simulink library "Collector_EN12975_FlatPlate_CONF"  (R2013b)
settings: Solver=ode45  StartTime=0.0  StopTime=10.0  RelTol=1e-3
undefined symbols (not defined in the file): FPC
libraries: carnot x2
settings Model: Creator=lena.frank  LastModifiedBy=drhf

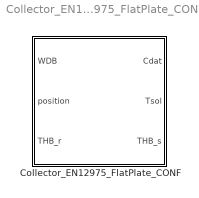
== system Collector_EN12975_FlatPlate_CONF ==
  Collector_EN12975_FlatPlate_CONF : Subsystem  mask(configurated Flat Plate Solar Thermal Collector){parameterfile=DefaultCollectorFlatPlate, tini=20, Ncollector=1}
      mask prompts: parameterfile "Parameter set"; tini "Inital temperature in °C"; Ncollector "Number of collectors in parallel"
      mask help:
      | Dynamic 1-node collector model according to EN 12975 standard using the b0 model for flat plate collector optics.
      | This block uses predefined parameter sets.
      mask init:
      | % path definitions
      | intpath = fullfile(path_carnot('intlibsl'), 'Source','Solar_Thermal', ...
      |     'Collector_EN12975_FlatPlate_CONF','parameter_set');
      | pubpath = fullfile(path_carnot('libsl'), 'Source','Solar_Thermal', ...
      |     'Collector_EN12975_FlatPlate_CONF','parameter_set');
      | 
      | [namelist, lib] = CarnotCallbacks_getConfNamelist(intpath,pubpath);
      | 
      | % set namelist in mask
      | if ~lib
      |     myMaskStylesVar{1} = ['popup(', namelist,')'];
      |     myMaskStylesVar{2} = 'edit';
      |     myMaskStylesVar{3} = 'edit';
      |     set_param(gcb, 'MaskStyles', myMaskStylesVar);
      | end
      | 
      | if exist(fullfile(intpath,[parameterfile '.mat']))
      |     load(fullfile(intpath,parameterfile));
      | else
      |     load(fullfile(pubpath,parameterfile));
      | end
      mask Help: web(fullfile(path_carnot('help'),'collector_en12975.html'),'-helpbrowser')
      mask TypeOptions parameterfile: DefaultCollectorFlatPlate | Vitosol100F_SV1A_2_5m2 | Vitosol200F_SV2A_2_5m2 | Vitosol200F_SV2B_2_5m2 | Vitosol200F_SV2C_2_5m2 | Vitosol300F_SV3C_2_5m2
      mask Display:
      | % user defined picture file
      | picfile = fullfile(path_carnot('intlibsl'), ...
      |     'Source','Solar_Thermal','Collector_EN12975_FlatPlate_CONF','parameter_set', ...
      |     'Collector_CONF.jpg');
      | 
      | pic = false;
      | 
      | % show internal picture if defined
      | if ~BlockIsInCarnotLibrary    % if not located in library any more
      |     if exist(picfile)
      |         image(imread(picfile), [0, 0, 1, 1])
      |         set_param(gcb, 'BackgroundColor', 'White')
      |         pic = true;
      |     end
      | end
      | 
      | if ~pic % show public picture
      |     set_param(gcb, 'BackgroundColor', 'Yellow')
      |     disp('solar thermal\ncollector\nEN 12975\nB0-Optics')
      | end
      | 
      | % Show port labels: same as port labels in the subsystem,
      | % but display with a picture covers the text. Have to reprint it.
      | port_label('input',1,'WDB')
      | port_label('input',2,'position')
      | port_label('input',3,'THB_r')
      | port_label('output',1,'Cdat')
      | port_label('output',2,'Tsol')
      | port_label('output',3,'THB_s')

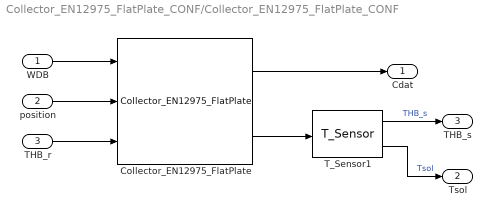
== system Collector_EN12975_FlatPlate_CONF/Collector_EN12975_FlatPlate_CONF ==
  WDB : Inport
  position : Inport  Port=2
  THB_r : Inport  Port=3
  Collector_EN12975_FlatPlate : carnot/Source/Solar_Thermal/Collector_EN12975_FlatPlate  acol=FPC.Acoll*Ncollector  len=FPC.len  fta=FPC.fta  c1=FPC.c1  c2=FPC.c2  c3=FPC.c3  c4=FPC.c4  c5=FPC.c5  c6=FPC.c6  b0=FPC.b0  Kd=FPC.Kd  lin=FPC.lin/Ncollector  qua=FPC.qua/(Ncollector^2)  tini=tini
  T_Sensor1 : carnot/Control/T_Sensor  tc=FPC.SensorTimeConstant  t0=tini
  Cdat : Outport
  Tsol : Outport  Port=2
  THB_s : Outport  Port=3
  wires:
  Collector_EN12975_FlatPlate/1 -> Cdat/1
  THB_r/1 -> Collector_EN12975_FlatPlate/3
  position/1 -> Collector_EN12975_FlatPlate/2
  WDB/1 -> Collector_EN12975_FlatPlate/1
  Collector_EN12975_FlatPlate/2 -> T_Sensor1/1
  T_Sensor1/1 -> THB_s/1  "THB_s"
  T_Sensor1/2 -> Tsol/1  "Tsol"
